simulink model "ADP_1LinkRobot_PEFree_ModFree"  (R2018b)
settings: Solver=ode1  StartTime=0.0  StopTime=10  FixedStep=1/1000  RelTol=1e-3  AbsTol=1e-3  EnableMultiTasking=on
PostLoadFcn:
  | f_Simulink_figureplace
InitFcn:
  | ADP_1LinkRobot_PEFree_ModFree_PreSim
values from neighbouring files (symbols this model uses):
  beta = 3    [ADP_1LinkRobot_PEFree_ModFree_PreSim.m]
  DY1 = 2    [ADP_1LinkRobot_PEFree_ModFree_PreSim.m]
  DY2 = 4    [ADP_1LinkRobot_PEFree_ModFree_PreSim.m]
  etaa1 = 10    [ADP_1LinkRobot_PEFree_ModFree_PreSim.m]
  etaa2 = 0.1    [ADP_1LinkRobot_PEFree_ModFree_PreSim.m]
  etac1 = 0.1    [ADP_1LinkRobot_PEFree_ModFree_PreSim.m]
  etac2 = 0.5    [ADP_1LinkRobot_PEFree_ModFree_PreSim.m]
  F = 9    [ADP_1LinkRobot_PEFree_ModFree_PreSim.m]
  fs = 1000    [ADP_1LinkRobot_PEFree_ModFree_PreSim.m]
  Gamma0 = 100*eye(L)    [ADP_1LinkRobot_PEFree_ModFree_PreSim.m]
  GammaBar = 100000    [ADP_1LinkRobot_PEFree_ModFree_PreSim.m]
  GammaTheta = diag([20 20 20 20])    [ADP_1LinkRobot_PEFree_ModFree_PreSim.m]
  GG = [GG;phi_pc*Gc*(R\Gc')*phi_pc']    [ADP_1LinkRobot_PEFree_ModFree_PreSim.m]
  k = 10    [ADP_1LinkRobot_PEFree_ModFree_PreSim.m]
  kTheta = 30    [ADP_1LinkRobot_PEFree_ModFree_PreSim.m]
  L = 3    [ADP_1LinkRobot_PEFree_ModFree_PreSim.m]
  learning = 1    [ADP_1LinkRobot_PEFree_ModFree_PreSim.m]
  M = 30    [ADP_1LinkRobot_PEFree_ModFree_PreSim.m]
  model = 0    [ADP_1LinkRobot_PEFree_ModFree_PreSim.m]
  N = length(Xc)^n    [ADP_1LinkRobot_PEFree_ModFree_PreSim.m]
  n = 2    [ADP_1LinkRobot_PEFree_ModFree_PreSim.m]
  pecutoff = 0.4    [ADP_1LinkRobot_PEFree_ModFree_PreSim.m]
  PHIPY = [PHIPY;phi_pc*Yc]    [ADP_1LinkRobot_PEFree_ModFree_PreSim.m]
  Q = [1 0 ; 0 1]    [ADP_1LinkRobot_PEFree_ModFree_PreSim.m]
  R = 1    [ADP_1LinkRobot_PEFree_ModFree_PreSim.m]
  theta0 = 1*[1; 1; 1; 1]    [ADP_1LinkRobot_PEFree_ModFree_PreSim.m]
  v = 0.005    [ADP_1LinkRobot_PEFree_ModFree_PreSim.m]
  WaH0 = 1*WcH0    [ADP_1LinkRobot_PEFree_ModFree_PreSim.m]
  WcH0 = 1*[1 1 1]'    [ADP_1LinkRobot_PEFree_ModFree_PreSim.m]
  x0 = [-1;-1]    [ADP_1LinkRobot_PEFree_ModFree_PreSim.m]
  XQX = zeros(N,1)    [ADP_1LinkRobot_PEFree_ModFree_PreSim.m]
undefined symbols (not defined in the file or in its folder): g
settings Model: Creator=rkamalapurkar  LastModifiedBy=rushik
settings SolverCC: AutoScaleAbsTol=off
settings DataIOCC: SaveFormat=StructureWithTime  SaveOutput=off  SaveTime=off
settings OptimizationCC: ExpressionDepthLimit=2147483647  LifeSpan=inf
settings DebuggingCC: UnderspecifiedInitializationDetection=Classic  MergeDetectMultiDrivingBlocksExec=none  SolverPrmCheckMsg=warning  FcnCallInpInsideContextMsg=warning  StateNameClashWarn=warning  SFUnexpectedBacktrackingDiag=warning  SFNoUnconditionalDefaultTransitionDiag=warning  SFExecutionAtInitializationDiag=none
settings HardwareCC: ProdBitPerPointer=32  ProdBitPerSizeT=32  ProdBitPerPtrDiffT=32  ProdLargestAtomicFloat=None  ProdIntDivRoundTo=Undefined  ProdEndianess=Unspecified  ProdWordSize=32  ProdHWDeviceType=32-bit Generic
settings ModelReferenceCC: PropagateSignalLabelsOutOfModel=off
settings SFSimCC: SimUseLocalCustomCode=off
settings RTWCC: RTWUseLocalCustomCode=off
settings CodeAppCC: StateflowObjectComments=on
settings GRTTargetCC: TargetLangStandard=C89/C90 (ANSI)  GeneratePreprocessorConditionals=Disable all  CombineOutputUpdateFcns=off  GRTInterface=on
settings ConfigComp: CovMetricSettings=dw  CovHtmlReporting=on  CovSaveCumulativeToWorkspaceVar=on  CovSaveSingleToWorkspaceVar=on  CovExternalEMLEnable=off  CovSFcnEnable=off

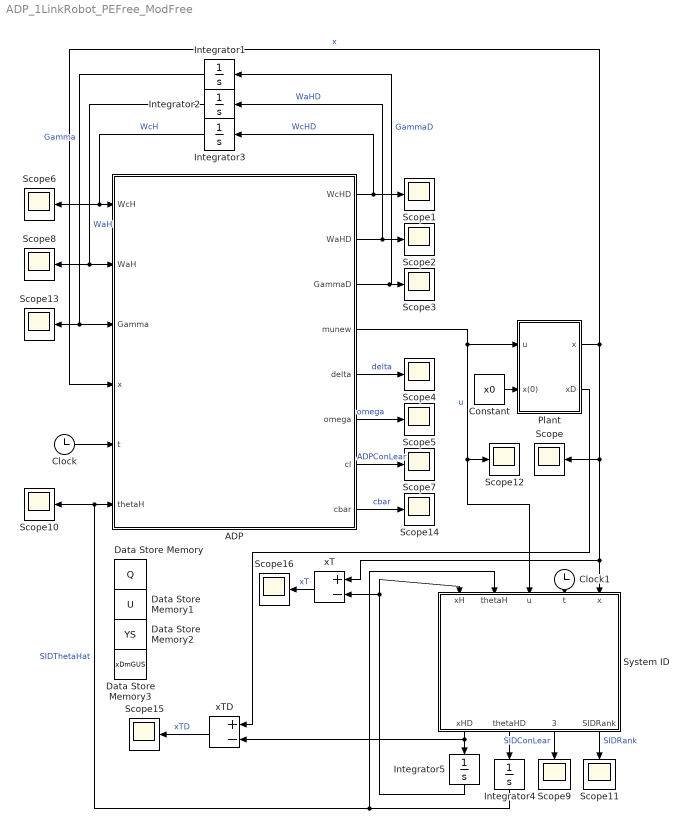
== system ADP_1LinkRobot_PEFree_ModFree ==
  ADP : MATLAB Function  TreatAsAtomicUnit=on
  Clock : Clock
  Clock1 : Clock
  Constant : Constant  Value=x0
  Data Store Memory : DataStoreMemory  DataStoreName=Q  InitialValue=zeros(n,F)  ShowAdditionalParam=off  OutDataTypeStr=double
  Data Store Memory1 : DataStoreMemory  DataStoreName=U  InitialValue=zeros(1,(F+1)/2)  ShowAdditionalParam=off  OutDataTypeStr=double
  Data Store Memory2 : DataStoreMemory  DataStoreName=YS  InitialValue=zeros(DY2,DY1*M)  ShowAdditionalParam=off  OutDataTypeStr=double
  Data Store Memory3 : DataStoreMemory  DataStoreName=xDmGUS  InitialValue=zeros(n,M)  ShowAdditionalParam=off  OutDataTypeStr=double
  Integrator1 : Integrator  InitialCondition=Gamma0
  Integrator2 : Integrator  InitialCondition=WaH0
  Integrator3 : Integrator  InitialCondition=WcH0
  Integrator4 : Integrator  InitialCondition=theta0
  Integrator5 : Integrator  InitialCondition=zeros(n,1)
  Plant : Subsystem
  Scope{,1..16} (17 alike) : Scope
  System ID : MATLAB Function  TreatAsAtomicUnit=on
  xT : Sum  Inputs=+-
  xTD : Sum  Inputs=+-
  wires:
  ADP/3(GammaD) -> Integrator1/1, Scope3/1  "GammaD"
  ADP/1(WcHD) -> Scope1/1, Integrator3/1  "WcHD"
  Integrator3/1 -> Scope6/1, ADP/1(WcH)  "WcH"
  ADP/2(WaHD) -> Integrator2/1, Scope2/1  "WaHD"
  Integrator2/1 -> ADP/2(WaH), Scope8/1  "WaH"
  ADP/5(delta) -> Scope4/1  "delta"
  ADP/6(omega) -> Scope5/1  "omega"
  Integrator1/1 -> Scope13/1, ADP/3(Gamma)  "Gamma"
  Clock/1 -> ADP/5(t)
  ADP/4(munew) -> System ID/3(u), Scope12/1, Plant/1(u)  "u"
  ADP/7(cl) -> Scope7/1  "ADPConLear"
  Integrator4/1 -> Scope10/1, ADP/6(thetaH), System ID/2(thetaH)  "SIDThetaHat"
  Plant/1(x) -> ADP/4(x), xT/1, System ID/5(x), Scope/1  "x"
  Constant/1 -> Plant/2(x(0))
  System ID/1(xHD) -> xTD/2, Integrator5/1
  Integrator5/1 -> xT/2, System ID/1(xH)
  System ID/4(SIDRank) -> Scope11/1  "SIDRank"
  System ID/3(SIDConLear) -> Scope9/1  "SIDConLear"
  System ID/2(thetaHD) -> Integrator4/1
  Clock1/1 -> System ID/4(t)
  ADP/8(cbar) -> Scope14/1  "cbar"
  Plant/2(xD) -> xTD/1
  xTD/1 -> Scope15/1  "xTD"
  xT/1 -> Scope16/1  "xT"

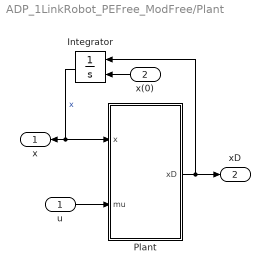
== system ADP_1LinkRobot_PEFree_ModFree/Plant ==
  u : Inport
  x(0) : Inport  Port=2
  Integrator : Integrator  InitialConditionSource=external  InitialCondition=[1;1;0.0;0.0]
  Plant : MATLAB Function  TreatAsAtomicUnit=on
  x : Outport
  xD : Outport  Port=2
  wires:
  Plant/1(xD) -> Integrator/1, xD/1
  Integrator/1 -> Plant/1(x), x/1  "x"
  u/1 -> Plant/2(mu)
  x(0)/1 -> Integrator/2

== matlab function ADP_1LinkRobot_PEFree_ModFree/Plant/Plant ==
  data: xD output; x input; mu input
function xD = dynamics(x,mu)
%#codegen
F=[-x(1)+x(2) ;-0.5*x(1)-0.5*x(2)*(1-(cos(2*x(1))+2)^2)];
G=[0; (cos(2*x(1))+2)];
xD = F+G*mu;

== matlab function ADP_1LinkRobot_PEFree_ModFree/ADP ==
  data: WcH input; WaH input; Gamma input; x input; t input; thetaH input; tf parameter; R parameter; Q parameter; etaa1 parameter; etaa2 parameter; etac1 parameter; etac2 parameter; v parameter; XQX parameter; GG parameter; PHIPY parameter; N parameter; pecutoff parameter; learning parameter; WcHD output; WaHD output; GammaD output; munew output; delta output; omega output; cl output; model parameter; L parameter; beta parameter; GammaBar parameter; cbar output
function [WcHD,WaHD,GammaD,munew,delta,omega,cl,cbar]=...
    control(WcH,WaH,Gamma,x,t,thetaH,tf,R,Q,etaa1,etaa2,...
    etac1,etac2,v,XQX,GG,PHIPY,N,pecutoff,learning,model,L,beta,GammaBar)
%#codegen
thetaS=[-1 1 -0.5 -0.5]'; % True values of SysID Parameters

G = [0 ; (cos(2*x(1))+2)];
Y = [x(1) x(2) 0 0;0 0 x(1) x(2)*(1-(cos(2*x(1))+2)^2)];

phi_p =[2*x(1) 0; x(2) x(1); 0 2*x(2)];

mu=-0.5*(R\G')*phi_p'*WaH;
% pe = sin(2*pi*t) + sin(exp(1)*t) + cos(5*t)^5 ;
pe = (sin(t)^2*cos(t)+sin(2*t)^2*cos(0.1*t)+sin(-1.2*t)^2*cos(0.5*t)+sin(t)^5);
munew = mu + pe*(t<=tf*pecutoff)*(learning==2);

theta = thetaS*(model==1) + thetaH*(model~=1);
%% Concurrent Learning

GGWaH = reshape(GG*WaH,L,N);
PHIPYtheta = reshape(PHIPY*theta,L,N);
deltac = (PHIPYtheta')*WcH + XQX-(1/2)*(GGWaH'*WcH)+(1/4)*(GGWaH'*WaH);
Omegac = (PHIPYtheta-(1/2)*(GGWaH));
normm=1./(1.+v.*dot(Omegac.',Omegac.'*Gamma.',2));
cbar = real(min(eig(Omegac*diag(normm)*Omegac')));
cl = (-etac2*Gamma*Omegac*diag(normm)*deltac/N)*(learning==1);

%% ADP
omega = phi_p*(Y*theta+G*mu);
Gsigma = phi_p*G*(R\G')*phi_p';
r = x'*Q*x + mu'*R*mu;
delta = WcH'*omega + r;
rho = (1+v*omega'*(Gamma)*omega);
WcHD = (-etac1*Gamma*omega*delta/rho+cl);
GammaD = (beta*Gamma-Gamma*(omega*omega'/rho^2)*Gamma)*(norm(Gamma)<=GammaBar);
WaHD = etaa1*(WcH-WaH)...
    +(-etaa2*WaH+etac1*Gsigma'*WaH*omega'*WcH/(4*rho))*(learning==1)...
    +(etac2*GGWaH*(Omegac*diag(normm))'*WcH/(4*N))*(learning==1);

== matlab function ADP_1LinkRobot_PEFree_ModFree/System ID ==
  settings: updateMethod=DISCRETE
  data: xH input; xHD output; thetaH input; thetaHD output; u input; SIDConLear output; SIDRank output; t input; x input; k parameter; GammaTheta parameter; M parameter; Q data_store_memory; fs parameter; F parameter; g parameter; YS data_store_memory; xDmGUS data_store_memory; U data_store_memory; DY1 parameter; kTheta parameter
function [xHD,thetaHD,SIDConLear,SIDRank] = SysID(xH,thetaH,u,t,x,k,...
    GammaTheta,M,fs,F,g,DY1,kTheta)
%#codegen
% This simulink block implements concurrent-learning based system
% identification using a Savitzky–Golay smoothing filter for state
% derivative computation. 
% fs: Sampling frequency
% M: number of stored data points
% F: Savitzky–Golay filter window length
% g: Savitzky–Golay filter differentiation matrix

global Q; % Data store memory for storing the values of x
global U; % Data store memory for storing the values of u
global YS; % Data store memory for storing the values of Y,
           % made of Y' matrices stacked in a row
global xDmGUS; % Data store memory for storing the values of xDot - G*u

n=round(t*fs)+1; % Current iteration number

xT = x-xH; % XTilde

%Dynamics
G = [0 ; cos(2*x(1))+2];
Y = [x(1) x(2) 0 0 ;0 0 x(1) x(2)*(1-(cos(2*x(1))+2)^2)];

% For the first M points, store the values of Y and G*u
if n<=M
    YS(:,DY1*n-(DY1-1):DY1*n)=Y';
    xDmGUS(:,n)=G*u; % This will be subtracted from xDot later.
end

% At every time n store the past F values of the state. Note that 
% Q*g(:,2)/(1/fs) gives the state derivative at n-(F-1)/2
if n<=F
    Q(:,n)=x;
else
    Q = [Q(:,2:F) x];
end

% At every time n store the past (F+1)/2 values of the control. Actually, 
% we only need the value of u at n-(F-1)/2. However, I could not find a way
% to store just that single value. Also, even if U is initialized as a row
% vector, MATLAB seems to think its a column.
if n<=(F+1)/2
    U(n)=u;
else
    U = [U(2:(F+1)/2); u];
end

% Since the state derivative information is only available if n>=F and at 
% each time n, we can compute the state derivative evaluated at time 
% n-(F-1)/2, at time M+(F-1)/2, we we can evaluate the values of the state
% derivative at time steps from F-(F-1)/2 to M. Which in turn means that at
% this point we have M-(F+1)/2 usable values of XDot - G*u in the data
% store xDnGUs. The first (F-1)/2 values in xDmGUS are not usable.

index=0; 
nSt = (F+1)/2; % This is the starting index of usable values (=1+(F-1)/2)
if n<=M+(F-1)/2
    if n>=F % 
        xDj=Q*g(:,2)/(1/fs); % This is the state derivative at n-(F-1)/2
        xDmGUS(:,(n-(F-1)/2))=xDj-xDmGUS(:,(n-(F-1)/2));
    end
else 
    
% When n>M+(F-1)/2, use singular value maximization algorithm to replace
% elements of YS and XDmGUS with new data. At each time n, the value of the 
% state at n-(F-1)/2 can be found in Q(:,(F+1)/2)
    xj=Q(:,(F+1)/2); 
    Yj = [xj(1) xj(2) 0 0;0 0 xj(1) xj(2)*(1-(cos(2*xj(1))+2)^2)];
    REGste1 = YS(:,DY1*nSt-(DY1-1):DY1*M)*YS(:,DY1*nSt-(DY1-1):DY1*M)';
    svd1=min(svd(REGste1)); % Minimum singular value of existing data
    for i=nSt:M
        te=YS; % Store existing data in a temporary variable
        te(:,DY1*i-(DY1-1):DY1*i)=Yj'; % Replac i'th Y' matrix with Yj'
        REGste2 = te(:,DY1*nSt-(DY1-1):DY1*M)*te(:,DY1*nSt-(DY1-1):DY1*M)';
        svd2=min(svd(REGste2)); % Minimum singular value after replacement
        if svd1<svd2   % If replacement results in a higher singular value,
            index=i;   % note the index of replacement and
            svd1=svd2; % keep searching for an even higher singular value.          
        end
    end
    
% At this point, index points to the matrix Y' in the stack YS which, when
% replaced with the new matrix Yj', results in the highest singular value.
% If index=0, the new data point is discarded. Otherwise, the stack YS, and
% correspondingly the stack xDmGUS is updated with the new data point. Note
% that since there is a delay of (F-1)/2 for derivative computation, the
% "new" data point we are talking about is the one that was recorded 
% (F-1)/2 steps ago.
    if index ~= 0
        YS(:,DY1*index-(DY1-1):DY1*index)=Yj';
        uj=U(1,1);
        xDj=Q*g(:,2)/(1/fs);
        Gj = [0 ; cos(2*xj(1))+2];
        xDmGUS(:,index)=xDj-Gj*uj;
    end
end

xHD = Y*thetaH + G*u + k*xT;

% Find the index nEn of the last usable data point. This is only relevent 
% when n <= M+(F-1)/2. Otherwise, nEn = M.
nEn = nSt;
if n<=M+(F-1)/2 && n>=F
    nEn = n-(F-1)/2;
elseif n>M+(F-1)/2
    nEn=M; 
end
nEn = min(nEn,M);

% Final computation for the concurrent learning-based component of the
% adaptive update law. The concurrent learning component is zero for the
% first F timesteps.
REGs = YS(:,DY1*nSt-(DY1-1):DY1*nEn)*YS(:,DY1*nSt-(DY1-1):DY1*nEn)'*(n>=F);
SIDRank = min(svd(REGs)); % For plots
REG1s = YS(:,DY1*nSt-(DY1-1):DY1*nEn)*...
    reshape(xDmGUS(:,nSt:nEn),DY1*(nEn-nSt+1),1)*(n>=F);
SIDConLear = (REG1s-REGs*thetaH)/(nEn-nSt+1);
thetaHD = 0*GammaTheta*Y'*xT + kTheta*GammaTheta*SIDConLear;
